simulink model "ac_checks_A_test"  (R2024b)
settings: Solver=ode45  StartTime=0.0  StopTime=200  RelTol=1e-3
PreLoadFcn:
  | load_system('../simulink_reference_models/test_sequence_lib');
InitFcn:
  | close all
  | clear all
  | 
  | T_CNTL = 1/5e3;
  | 
  | VLL_NOM = 35e3;
  | F_NOM = 60;
libraries: test_sequence_lib x5
settings Model: SimulationMode=rapid-accelerator  Creator=HussamAlatrash  LastModifiedBy=ritvik_heron

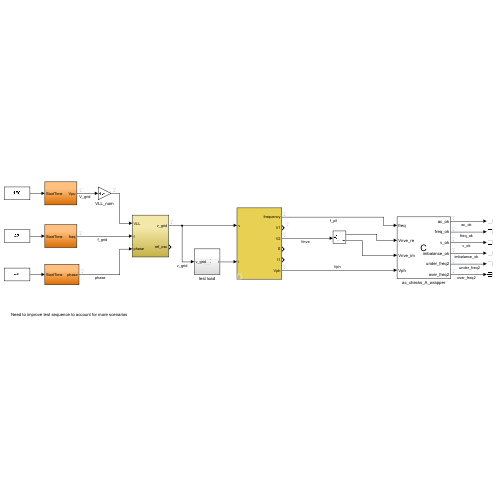
[thumbnail: Simulink's stored preview of the top-level diagram]
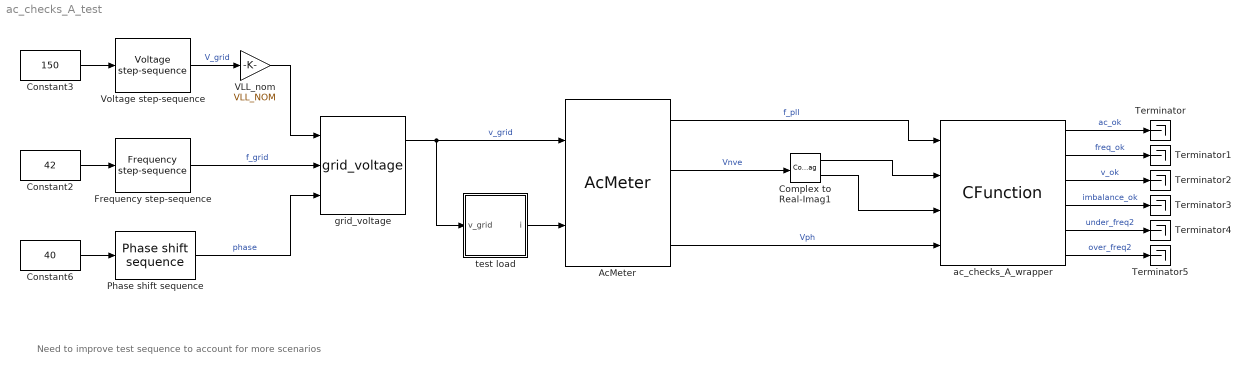
== system ac_checks_A_test ==
  note: Need to improve test sequence to account for more scenarios
  AcMeter : test_sequence_lib/AcMeter  VllRated=VLL_NOM
  Complex to Real-Imag1 : ComplexToRealImag
  Constant2 : Constant  Value=42
  Constant3 : Constant  Value=150
  Constant6 : Constant  Value=40
  Frequency step-sequence : test_sequence_lib/Frequency step-sequence  SystemSampleTime=-1  VariantActivationTime=update diagram  AllowFlexibleInterface=on  Latency=0  AutoFrameSizeCalculation=off
  Phase shift sequence : test_sequence_lib/Phase shift sequence  SystemSampleTime=-1  VariantActivationTime=update diagram  AllowFlexibleInterface=on  Latency=0  AutoFrameSizeCalculation=off
  Terminator{,1..5} (6 alike) : Terminator
  VLL_nom : Gain  Gain=VLL_NOM
  Voltage step-sequence : test_sequence_lib/Voltage step-sequence  SystemSampleTime=-1  VariantActivationTime=update diagram  AllowFlexibleInterface=on  Latency=0  AutoFrameSizeCalculation=off
  ac_checks_A_wrapper : CFunction  OutputCode=|  StartCode=|  CodegenOutputCode=|  CodegenStartCode=|  SampleTime=1e-3  SimCustomHeaderFile=../c_language_library/companion_algorithms/ac_checks_A/acChecks_A_autogen.h  SimCustomSourceFile=|  CustomHeaderFile=../c_language_library/companion_algorithms/ac_checks_A/acChecks_A_autogen.h  CustomSourceFile=|
      OutputCode=|
      | acChecks_IN.freq = freq;
      | acChecks_IN.Vnve.real = Vnve_re;
      | acChecks_IN.Vnve.imag = Vnve_im;
      | 
      | uint16_t i;
      | for (i = 0; i < 3; i++) 
      | {
      |     acChecks_IN.Vph[i] = Vph[i];
      | }
      | 
      | acChecks_1kHz(1e-3f);
      | 
      | ac_ok = acChecks_OUT.acOk;
      | freq_ok = acChecks_QUALIFY_STATE.freqInrange;
      | v_ok = acChecks_QUALIFY_STATE.voltageInrange;
      | imbalance_ok = acChecks_QUALIFY_STATE.vimbalanceInrange;
      | 
      | under_freq2 = acChecks_TRIP_STATE.underFrequency2State;
      | over_freq2 = acChecks_TRIP_STATE.overFrequency2State;
      StartCode=|
      | set_acChecks_GENERAL_CFG_VllRated(35e3);
      | acChecks_update_derived_config();
      CodegenOutputCode=|
      | acChecks_IN.freq = freq;
      | acChecks_IN.Vnve.real = Vnve_re;
      | acChecks_IN.Vnve.imag = Vnve_im;
      | 
      | uint16_t i;
      | for (i = 0; i < 3; i++) 
      | {
      |     acChecks_IN.Vph[i] = Vph[i];
      | }
      | 
      | acChecks_1kHz(1e-3f);
      | 
      | ac_ok = acChecks_OUT.acOk;
      | freq_ok = acChecks_QUALIFY_STATE.freqInrange;
      | v_ok = acChecks_QUALIFY_STATE.voltageInrange;
      | imbalance_ok = acChecks_QUALIFY_STATE.vimbalanceInrange;
      | 
      | under_freq2 = acChecks_TRIP_STATE.underFrequency2State;
      | over_freq2 = acChecks_TRIP_STATE.overFrequency2State;
      CodegenStartCode=|
      | set_acChecks_GENERAL_CFG_VllRated(35e3);
      | acChecks_update_derived_config();
      SimCustomSourceFile=|
      | ../c_language_library/companion_algorithms/ac_checks_A/ac_checks_A.c
      | ../c_language_library/helper_lib/timers.c
      | ../c_language_library/helper_lib/cmplx.c
      CustomSourceFile=|
      | ../c_language_library/companion_algorithms/ac_checks_A/ac_checks_A.c
      | ../c_language_library/helper_lib/timers.c
      | ../c_language_library/helper_lib/cmplx.c
  grid_voltage : test_sequence_lib/grid_voltage  SystemSampleTime=-1  VariantActivationTime=update diagram  AllowFlexibleInterface=on  Latency=0  AutoFrameSizeCalculation=off
  test load : Subsystem
  wires:
  VLL_nom/1 -> grid_voltage/1
  Phase shift sequence/1 -> grid_voltage/3  "phase"
  Voltage step-sequence/1 -> VLL_nom/1  "V_grid"
  Constant3/1 -> Voltage step-sequence/1
  Frequency step-sequence/1 -> grid_voltage/2  "f_grid"
  Constant2/1 -> Frequency step-sequence/1
  Constant6/1 -> Phase shift sequence/1
  grid_voltage/1 -> AcMeter/1, test load/1(v_grid)  "v_grid"
  test load/1(i) -> AcMeter/2
  AcMeter/1 -> ac_checks_A_wrapper/1  "f_pll"
  ac_checks_A_wrapper/2 -> Terminator1/1  "freq_ok"
  ac_checks_A_wrapper/1 -> Terminator/1  "ac_ok"
  ac_checks_A_wrapper/3 -> Terminator2/1  "v_ok"
  ac_checks_A_wrapper/4 -> Terminator3/1  "imbalance_ok"
  ac_checks_A_wrapper/5 -> Terminator4/1  "under_freq2"
  ac_checks_A_wrapper/6 -> Terminator5/1  "over_freq2"
  Complex to Real-Imag1/1 -> ac_checks_A_wrapper/2
  Complex to Real-Imag1/2 -> ac_checks_A_wrapper/3
  AcMeter/3 -> Complex to Real-Imag1/1  "Vnve"
  AcMeter/6 -> ac_checks_A_wrapper/4  "Vph"

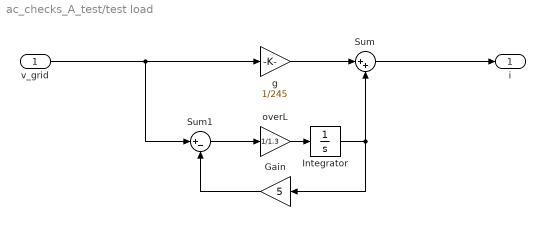
== system ac_checks_A_test/test load ==
  v_grid : Inport
  Gain : Gain  Gain=5
  Integrator : Integrator
  Sum : Sum  Inputs=|++
  Sum1 : Sum  Inputs=|+-
  g : Gain  Gain=1/245
  overL : Gain  Gain=1/1.3
  i : Outport
  wires:
  v_grid/1 -> g/1, Sum1/1
  overL/1 -> Integrator/1
  Integrator/1 -> Gain/1, Sum/2
  Sum1/1 -> overL/1
  Sum/1 -> i/1
  g/1 -> Sum/1
  Gain/1 -> Sum1/2
